simulink model "FullModelAddANN_Final_ANN_revised"  (R2024b)
settings: Solver=ode4  StartTime=0.0  StopTime=40  FixedStep=1e-5  RelTol=1e-3
values from neighbouring files (symbols this model uses):
  Dp = 2.506338228783948e3    (= 2506.33822878)    [FullModelAddANNm_Final.m]    (also in main_opal_ann_control.m)
  Dq = 1.033099625954584    (= 1.03309962595)    [FullModelAddANNm_Final.m]    (also in main_opal_ann_control.m)
  Kp = 0.006383815167581    (= 0.00638381516758)    [FullModelAddANNm_Final.m]    (also in main_opal_ann_control.m)
  Kq = 0.076670166944346    (= 0.0766701669443)    [FullModelAddANNm_Final.m]    (also in main_opal_ann_control.m)
undefined symbols (not defined in the file or in its folder): Filter, Ls, params
libraries: neural x88, spsCurrentMeasurementLib x6, spsParallelRLCBranchLib x6, spsIGBTDiodeLib x6, spsMeanLib x6, spsSeriesRLCBranchLib x6, simulink x4, spsVoltageMeasurementLib x4, spsVariableInductorLib x3, spsVariableResistorLib x3, spsDCVoltageSourceLib x1, spsThreePhaseSourceLib x1
(part 2 of 11)

== system FullModelAddANN_Final_ANN_revised/Feed-Forward Neural Network2/Process Output 1 ==
  a : Inport  PortDimensions=2
      mask Display: e = 0.06;c1 = [120 230 180]/255;c2 = ([120 230 180]+0)/(256+128);c3 = ([120 230 180]+128)/(256+128);patch([0 1 1 0],[0 0 1 1],c1);patch([0 1 1 1-e 1-e 0+e],[0 0 1 1-e 0+e 0+e],c2);patch([0 0 1 1-e 0+e 0+e],[0 1 1 1-e 1-e 0+e],c3);plot([0 1 1 0 0],[0 0 1 1 0]);
  mapminmax_reverse : neural/Processing Functions/mapminmax_reverse  xmin=[4.08518999999999987693399816635;0.100678000000000003599787135045]  xmax=[5.76843000000000039051428757375;1.28340000000000009627854069549]  ymin=-1  ymax=1
  y : Outport  PortDimensions=2
      mask Display: e = 0.06;c1 = [120 230 180]/255;c2 = ([120 230 180]+0)/(256+128);c3 = ([120 230 180]+128)/(256+128);patch([0 1 1 0],[0 0 1 1],c1);patch([0 1 1 1-e 1-e 0+e],[0 0 1 1-e 0+e 0+e],c2);patch([0 0 1 1-e 0+e 0+e],[0 1 1 1-e 1-e 0+e],c3);plot([0 1 1 0 0],[0 0 1 1 0]);
  wires:
  a/1 -> mapminmax_reverse/1
  mapminmax_reverse/1 -> y/1

== system FullModelAddANN_Final_ANN_revised/Feed-Forward Neural Network_Full/Layer 1 ==
  "p{1}" : Inport  PortDimensions=200
      mask Display: e = 0.06;c1 = [120 230 180]/255;c2 = ([120 230 180]+0)/(256+128);c3 = ([120 230 180]+128)/(256+128);patch([0 1 1 0],[0 0 1 1],c1);patch([0 1 1 1-e 1-e 0+e],[0 0 1 1-e 0+e 0+e],c2);patch([0 0 1 1-e 0+e 0+e],[0 1 1 1-e 1-e 0+e],c3);plot([0 1 1 0 0],[0 0 1 1 0]);
  Delays 1 : Subsystem
      mask Display: e = 0.06;c1 = [120 150 230]/255;c2 = ([120 150 230]+0)/383;c3 = ([120 150 230]+128)/383;patch([0 1 1 0],[0 0 1 1],c1);patch([0 1 1 1-e 1-e 0+e],[0 0 1 1-e 0+e 0+e],c2);patch([0 0 1 1-e 0+e 0+e],[0 1 1 1-e 1-e 0+e],c3);plot([0 1 1 0 0],[0 0 1 1 0]);disp('0');
  "IW{1,1}" : Subsystem
      mask Display: e = 0.06;c1 = [120 150 230]/255;c2 = ([120 150 230]+0)/383;c3 = ([120 150 230]+128)/383;patch([0 1 1 0],[0 0 1 1],c1);patch([0 1 1 1-e 1-e 0+e],[0 0 1 1-e 0+e 0+e],c2);patch([0 0 1 1-e 0+e 0+e],[0 1 1 1-e 1-e 0+e],c3);plot([0 1 1 0 0],[0 0 1 1 0]);disp('W');
  "b{1}" : Constant  Value=[-0.93745313626118720318203259012079797685146331787109375;-0.7522463014983509221877966410829685628414154052734375;0.7498310632798836916634854787844233214855194091796875;-0.448821782444379480114804437107522971928119659423828125;-0.56470000582433976799023866988136433064937591552734375;0.70695959761237425755808772009913809597492218017578125;0.305040499016989041791703130002133548259735107421875;0.045185602594992213543179104817681945860385894775390625;-0.385773129555622151798388586030341684818267822265625;0.402441364255973377250796829684986732900142669677734375;-0.458845318832768411798639363041729666292667388916015625;0.622328519648508216022264605271629989147186279296875;0.608199419849972944263072349713183939456939697265625;-0.7645386765801076567328209421248175203800201416015625;0.8420689862326191654773310801829211413860321044921875;-0.970352913386824500463490039692260324954986572265625]
      mask Display: e = 0.06;c1 = [120 150 230]/255;c2 = ([120 150 230]+0)/383;c3 = ([120 150 230]+128)/383;patch([0 1 1 0],[0 0 1 1],c1);patch([0 1 1 1-e 1-e 0+e],[0 0 1 1-e 0+e 0+e],c2);patch([0 0 1 1-e 0+e 0+e],[0 1 1 1-e 1-e 0+e],c3);plot([0 1 1 0 0],[0 0 1 1 0]);disp('b');
  netsum : Sum  Inputs=2  InputSameDT=on  SaturateOnIntegerOverflow=on  OutDataTypeStr=Inherit: Same as first input
      mask Display: e = 0.06;c1 = [120 150 230]/255;c2 = ([120 150 230]+0)/383;c3 = ([120 150 230]+128)/383;patch([0 1 1 0],[0 0 1 1],c1);patch([0 1 1 1-e 1-e 0+e],[0 0 1 1-e 0+e 0+e],c2);patch([0 0 1 1-e 0+e 0+e],[0 1 1 1-e 1-e 0+e],c3);plot([0 1 1 0 0],[0 0 1 1 0]);disp('+');
  tansig : neural/Transfer Functions/tansig
  "a{1}" : Outport  InitialOutput=[0;0;0;0;0;0;0;0;0;0;0;0;0;0;0;0]
      mask Display: e = 0.06;c1 = [120 230 180]/255;c2 = ([120 230 180]+0)/(256+128);c3 = ([120 230 180]+128)/(256+128);patch([0 1 1 0],[0 0 1 1],c1);patch([0 1 1 1-e 1-e 0+e],[0 0 1 1-e 0+e 0+e],c2);patch([0 0 1 1-e 0+e 0+e],[0 1 1 1-e 1-e 0+e],c3);plot([0 1 1 0 0],[0 0 1 1 0]);
  wires:
  "p{1}"/1 -> Delays 1/1("p{1}")
  Delays 1/1("pd{1,1}") -> "IW{1,1}"/1("pd{1,1}")
  "IW{1,1}"/1("iz{1,1}") -> netsum/1
  "b{1}"/1 -> netsum/2
  netsum/1 -> tansig/1
  tansig/1 -> "a{1}"/1

== system FullModelAddANN_Final_ANN_revised/Feed-Forward Neural Network_Full/Layer 2 ==
  "a{1} " : Inport  PortDimensions=16
      mask Display: e = 0.06;c1 = [120 230 180]/255;c2 = ([120 230 180]+0)/(256+128);c3 = ([120 230 180]+128)/(256+128);patch([0 1 1 0],[0 0 1 1],c1);patch([0 1 1 1-e 1-e 0+e],[0 0 1 1-e 0+e 0+e],c2);patch([0 0 1 1-e 0+e 0+e],[0 1 1 1-e 1-e 0+e],c3);plot([0 1 1 0 0],[0 0 1 1 0]);
  Delays 1 : Subsystem
      mask Display: e = 0.06;c1 = [120 150 230]/255;c2 = ([120 150 230]+0)/383;c3 = ([120 150 230]+128)/383;patch([0 1 1 0],[0 0 1 1],c1);patch([0 1 1 1-e 1-e 0+e],[0 0 1 1-e 0+e 0+e],c2);patch([0 0 1 1-e 0+e 0+e],[0 1 1 1-e 1-e 0+e],c3);plot([0 1 1 0 0],[0 0 1 1 0]);disp('0');
  "LW{2,1}" : Subsystem
      mask Display: e = 0.06;c1 = [120 150 230]/255;c2 = ([120 150 230]+0)/383;c3 = ([120 150 230]+128)/383;patch([0 1 1 0],[0 0 1 1],c1);patch([0 1 1 1-e 1-e 0+e],[0 0 1 1-e 0+e 0+e],c2);patch([0 0 1 1-e 0+e 0+e],[0 1 1 1-e 1-e 0+e],c3);plot([0 1 1 0 0],[0 0 1 1 0]);disp('W');
  "b{2}" : Constant  Value=[-0.349660820238201441867431640275754034519195556640625;0.1124855051162063634961896241293288767337799072265625]
      mask Display: e = 0.06;c1 = [120 150 230]/255;c2 = ([120 150 230]+0)/383;c3 = ([120 150 230]+128)/383;patch([0 1 1 0],[0 0 1 1],c1);patch([0 1 1 1-e 1-e 0+e],[0 0 1 1-e 0+e 0+e],c2);patch([0 0 1 1-e 0+e 0+e],[0 1 1 1-e 1-e 0+e],c3);plot([0 1 1 0 0],[0 0 1 1 0]);disp('b');
  netsum : Sum  Inputs=2  InputSameDT=on  SaturateOnIntegerOverflow=on  OutDataTypeStr=Inherit: Same as first input
      mask Display: e = 0.06;c1 = [120 150 230]/255;c2 = ([120 150 230]+0)/383;c3 = ([120 150 230]+128)/383;patch([0 1 1 0],[0 0 1 1],c1);patch([0 1 1 1-e 1-e 0+e],[0 0 1 1-e 0+e 0+e],c2);patch([0 0 1 1-e 0+e 0+e],[0 1 1 1-e 1-e 0+e],c3);plot([0 1 1 0 0],[0 0 1 1 0]);disp('+');
  purelin : neural/Transfer Functions/purelin
  "a{2}" : Outport  InitialOutput=[0;0]
      mask Display: e = 0.06;c1 = [120 230 180]/255;c2 = ([120 230 180]+0)/(256+128);c3 = ([120 230 180]+128)/(256+128);patch([0 1 1 0],[0 0 1 1],c1);patch([0 1 1 1-e 1-e 0+e],[0 0 1 1-e 0+e 0+e],c2);patch([0 0 1 1-e 0+e 0+e],[0 1 1 1-e 1-e 0+e],c3);plot([0 1 1 0 0],[0 0 1 1 0]);
  wires:
  "a{1} "/1 -> Delays 1/1("p{2}")
  Delays 1/1("pd{2,1}") -> "LW{2,1}"/1("ad{2,1}")
  "LW{2,1}"/1("lz{2,1}") -> netsum/1
  "b{2}"/1 -> netsum/2
  netsum/1 -> purelin/1
  purelin/1 -> "a{2}"/1

== system FullModelAddANN_Final_ANN_revised/Feed-Forward Neural Network_Full/Process Input 1 ==
  x : Inport  PortDimensions=200
      mask Display: e = 0.06;c1 = [120 230 180]/255;c2 = ([120 230 180]+0)/(256+128);c3 = ([120 230 180]+128)/(256+128);patch([0 1 1 0],[0 0 1 1],c1);patch([0 1 1 1-e 1-e 0+e],[0 0 1 1-e 0+e 0+e],c2);patch([0 0 1 1-e 0+e 0+e],[0 1 1 1-e 1-e 0+e],c3);plot([0 1 1 0 0],[0 0 1 1 0]);
  mapminmax : neural/Processing Functions/mapminmax  xmin=[-18.1541999999999994486188370502;-7.44869999999999965467623042059;3.20396999999999998465227690758;15.3264999999999993463006831007;26.545400000000000773070496507;39.4832999999999998408384271897;51.2171999999999982833287504036;62.2657999999999987039700499736;74.1317999999999983629095368087;85.9979000000000013415046851151;90.0867999999999966576069709845;84.7300000000000039790393202566;79.158100000000004570210876409;71.0503999999999962255969876423;70.2383999999999986130205797963;63.514400000000001966782292584;53.7342000000000012960299500264;49.1422999999999987608134688344;37.9063000000000016598278307356;33.1124999999999971578290569596;24.1713999999999984424903232139;20.1130999999999993121946317842;18.4002000000000016655121726217;7.66408000000000022566837287741;0.2774440000000000239310793404;-7.13638999999999956713736537495;-7.5049000000000001264766069653;-11.9069000000000002614797267597;-24.4015999999999984026999300113;-28.9071999999999995623056747718;-36.3990999999999971237230056431;-44.7280000000000015347723092418;-51.1516000000000019554136088118;-60.0354999999999989768184605055;-67.1332000000000022055246517994;-72.0875000000000056843418860808;-72.9534000000000020236257114448;-78.9898000000000024556356947869;-86.867500000000006821210263297;-90.046999999999997044142219238;-95.992500000000006821210263297;-96.6642999999999972260411595926;-100.924000000000006593836587854;-100.814999999999997726263245568;-103.352999999999994429344951641;-106.415000000000006252776074689;-105.480000000000003979039320257;-108.036000000000001364242052659;-108.385999999999995679900166579;-113.061999999999997612576407846;-113.593999999999994088284438476;-113.680999999999997385202732403;-113.947999999999993292476574425;-117.102999999999994429344951641;-118.498000000000004661160346586;-126.837000000000003296918293927;-137.923000000000001818989403546;-145.596000000000003637978807092;-149.325999999999993406163412146;-160.45699999999999363353708759;-169.43899999999999295141606126;-170.971000000000003637978807092;-175.950999999999993406163412146;-177.468999999999994088284438476;-177.054000000000002046363078989;-193.711999999999989086063578725;-190.943999999999988403942552395;-200.5;-204.413000000000010913936421275;-206.586999999999989086063578725;-212.259999999999990905052982271;-214.850999999999999090505298227;-215.110000000000013642420526594;-219.927999999999997271515894681;-213.552999999999997271515894681;-210.719999999999998863131622784;-204.14300000000000068212102633;-199.899000000000000909494701773;-194.169000000000011141310096718;-190.197000000000002728484105319;-187.044999999999987494447850622;-184.040999999999996816768543795;-184.417000000000001591615728103;-181.421999999999997044142219238;-173.832999999999998408384271897;-167.014999999999986357579473406;-159.828000000000002955857780762;-144.580000000000012505552149378;-132.871000000000009322320693173;-122.415999999999996816768543795;-110.460999999999998522071109619;-92.6098000000000070031092036515;-79.2937000000000011823431123048;-66.6076000000000050249582272954;-55.4363000000000027966962079518;-46.4945999999999983742782205809;-40.2008999999999971919351082761;-30.580400000000000915179043659;-26.3471000000000010743406164693;-23.6697999999999986187049216824;-12.1233000000000004092726157978;-12.2150999999999996248334355187;-12.7461999999999999744204615126;-12.8681000000000000937916411203;-13.8106000000000008753886504564;-13.5084999999999997299937604112;-12.3736999999999994770405464806;-11.4261999999999996902033672086;-10.8213000000000008071765478235;-9.86029000000000088732576841721;-8.03398999999999929855221125763;-5.84081000000000027938540370087;-4.18013999999999974477304931497;-2.83502000000000009549694368616;-1.46507999999999993789856489457;0.335683999999999982399856435222;1.85640000000000005009326287109;3.5641500000000001513456027169;4.22681000000000040017766878009;2.03202000000000015944578990457;-0.313620999999999983121057312019;-2.61730000000000018189894035459;-5.01956999999999986528109729989 ...(+2532 chars)]  xmax=[112.79999999999999715782905696;111.144999999999996020960679743;115.558000000000006934897101019;117.849000000000003751665644813;122.192999999999997839950083289;127.019999999999996020960679743;136.147999999999996134647517465;144.45699999999999363353708759;152.650000000000005684341886081;158.165999999999996816768543795;164.931000000000011596057447605;171.423000000000001818989403546;174.419999999999987494447850622;175.741000000000013869794202037;178.253999999999990677679306827;190.344999999999998863131622784;192.007000000000005002220859751;203.405000000000001136868377216;200.974999999999994315658113919;205.979999999999989768184605055;214.807999999999992724042385817;214.694999999999993178789736703;213.953000000000002955857780762;217.332999999999998408384271897;213;210.046999999999997044142219238;206.548000000000001818989403546;199.008000000000009777068044059;193.161000000000001364242052659;190.629999999999995452526491135;186.881000000000000227373675443;185.817000000000007275957614183;183.401999999999986812326824293;181.348999999999989540810929611;175.411000000000001364242052659;167.467000000000012960299500264;165.415999999999996816768543795;147.104999999999989768184605055;132.336999999999989086063578725;119.719999999999998863131622784;106.367000000000004433786671143;94.7475000000000022737367544323;78.5541000000000053660187404603;66.109499999999997044142219238;55.6694000000000031036506698001;47.8620999999999980900611262769;39.058199999999999363353708759;31.5702999999999995850430423161;27.5088000000000008071765478235;22.4850999999999991985077940626;14.745699999999999363353708759;6.72907999999999972828845784534;-2.79722999999999988318677424104;-15.5510000000000001563194018672;-25.9831000000000003069544618484;-39.7043000000000034788172342815;-51.9249000000000009436007530894;-62.2948999999999983856469043531;-74.8230999999999966121322358958;-85.0691999999999950432538753375;-81.6354000000000041836756281555;-79.7052999999999940428097033873;-75.7283000000000043883119360544;-65.9572000000000002728484105319;-60.3667999999999977944753482006;-55.1897999999999981923792802263;-49.7203999999999979308995534666;-43.0686999999999997612576407846;-38.2561999999999997612576407846;-31.8615999999999992553512129234;-26.1017000000000010118128557224;-20.3201000000000000511590769747;-13.9556000000000004490630090004;-3.78928000000000020364154806884;0.792328000000000032265745630866;8.75453000000000081115558714373;12.4443999999999999062083588797;12.5769000000000001904254531837;25.1676999999999999602096067974;30.4983000000000004092726157978;41.3939999999999983515408530366;49.8380000000000009663381206337;54.6548000000000016029844118748;61.4352000000000018076207197737;68.6329000000000064574123825878;77.1235999999999961573848850094;84.3909000000000020236257114448;87.9608999999999952024154481478;90.2530000000000001136868377216;95.6707999999999998408384271897;96.7533999999999991814547684044;99.2844999999999942019712761976;101.617999999999994997779140249;102.167000000000001591615728103;106.757000000000005002220859751;111.489999999999994884092302527;110.766000000000005343281372916;113.855999999999994543031789362;113.308999999999997498889570124;112.527000000000001023181539495;52.6158000000000001250555214938;51.8245000000000004547473508865;50.9217000000000012960299500264;49.8179000000000016257217794191;48.5294999999999987494447850622;47.0690999999999988290255714674;45.4183000000000021145751816221;43.5947999999999993292476574425;41.6131999999999990791366144549;39.4806000000000025806912162807;37.1856000000000008753886504564;37.7886999999999986243892635684;38.4459000000000017394086171407;38.670400000000000773070496507;38.4410000000000025011104298756;38.3459000000000003183231456205;38.2884000000000028762769943569;37.8397000000000005570655048359;36.9037999999999968281372275669;35.9100999999999999090505298227;34.9179000000000030468072509393;33.7860000000000013642420526594;32.5932999999999992724042385817;31.6207999999999991302956914296;30.511500000000001620037437533 ...(+2402 chars)]  ymin=-1  ymax=1
  p : Outport  PortDimensions=200
      mask Display: e = 0.06;c1 = [120 230 180]/255;c2 = ([120 230 180]+0)/(256+128);c3 = ([120 230 180]+128)/(256+128);patch([0 1 1 0],[0 0 1 1],c1);patch([0 1 1 1-e 1-e 0+e],[0 0 1 1-e 0+e 0+e],c2);patch([0 0 1 1-e 0+e 0+e],[0 1 1 1-e 1-e 0+e],c3);plot([0 1 1 0 0],[0 0 1 1 0]);
  wires:
  x/1 -> mapminmax/1
  mapminmax/1 -> p/1

== system FullModelAddANN_Final_ANN_revised/Feed-Forward Neural Network_Full/Process Output 1 ==
  a : Inport  PortDimensions=2
      mask Display: e = 0.06;c1 = [120 230 180]/255;c2 = ([120 230 180]+0)/(256+128);c3 = ([120 230 180]+128)/(256+128);patch([0 1 1 0],[0 0 1 1],c1);patch([0 1 1 1-e 1-e 0+e],[0 0 1 1-e 0+e 0+e],c2);patch([0 0 1 1-e 0+e 0+e],[0 1 1 1-e 1-e 0+e],c3);plot([0 1 1 0 0],[0 0 1 1 0]);
  mapminmax_reverse : neural/Processing Functions/mapminmax_reverse  xmin=[1.08938000000000001499245172454;0.0344836000000000031384672638524]  xmax=[11.5252999999999996560973158921;2.56680000000000019255708139099]  ymin=-1  ymax=1
  y : Outport  PortDimensions=2
      mask Display: e = 0.06;c1 = [120 230 180]/255;c2 = ([120 230 180]+0)/(256+128);c3 = ([120 230 180]+128)/(256+128);patch([0 1 1 0],[0 0 1 1],c1);patch([0 1 1 1-e 1-e 0+e],[0 0 1 1-e 0+e 0+e],c2);patch([0 0 1 1-e 0+e 0+e],[0 1 1 1-e 1-e 0+e],c3);plot([0 1 1 0 0],[0 0 1 1 0]);
  wires:
  a/1 -> mapminmax_reverse/1
  mapminmax_reverse/1 -> y/1

== system FullModelAddANN_Final_ANN_revised/Feed-Forward Neural Network_RealTime/Layer 1 ==
  "p{1}" : Inport  PortDimensions=200
      mask Display: e = 0.06;c1 = [120 230 180]/255;c2 = ([120 230 180]+0)/(256+128);c3 = ([120 230 180]+128)/(256+128);patch([0 1 1 0],[0 0 1 1],c1);patch([0 1 1 1-e 1-e 0+e],[0 0 1 1-e 0+e 0+e],c2);patch([0 0 1 1-e 0+e 0+e],[0 1 1 1-e 1-e 0+e],c3);plot([0 1 1 0 0],[0 0 1 1 0]);
  Delays 1 : Subsystem
      mask Display: e = 0.06;c1 = [120 150 230]/255;c2 = ([120 150 230]+0)/383;c3 = ([120 150 230]+128)/383;patch([0 1 1 0],[0 0 1 1],c1);patch([0 1 1 1-e 1-e 0+e],[0 0 1 1-e 0+e 0+e],c2);patch([0 0 1 1-e 0+e 0+e],[0 1 1 1-e 1-e 0+e],c3);plot([0 1 1 0 0],[0 0 1 1 0]);disp('0');
  "IW{1,1}" : Subsystem
      mask Display: e = 0.06;c1 = [120 150 230]/255;c2 = ([120 150 230]+0)/383;c3 = ([120 150 230]+128)/383;patch([0 1 1 0],[0 0 1 1],c1);patch([0 1 1 1-e 1-e 0+e],[0 0 1 1-e 0+e 0+e],c2);patch([0 0 1 1-e 0+e 0+e],[0 1 1 1-e 1-e 0+e],c3);plot([0 1 1 0 0],[0 0 1 1 0]);disp('W');
  "b{1}" : Constant  Value=[-0.7049546789635818822006285699899308383464813232421875;-0.53176379998661749137767174033797346055507659912109375;0.56664598808941513130577050105785019695758819580078125;-0.1546177681597955544390288196154870092868804931640625;-0.2268178266264400944063339693457237444818019866943359375;0.222921193941614304012688307921052910387516021728515625;0.139048173582270673254157600240432657301425933837890625;-0.1366552484170819592446122214823844842612743377685546875;0.0964330208189879412028489014119259081780910491943359375;-0.04916039248471136546836390834869234822690486907958984375;-0.7305750372192016950378956607892177999019622802734375;-0.1797210239748362747835841446431004442274570465087890625;0.45485073167759104695306859866832382977008819580078125;-0.475714928798503411400133700226433575153350830078125;0.77984233044243456145494519660132937133312225341796875;-0.73985496629634706078348926894250325858592987060546875]
      mask Display: e = 0.06;c1 = [120 150 230]/255;c2 = ([120 150 230]+0)/383;c3 = ([120 150 230]+128)/383;patch([0 1 1 0],[0 0 1 1],c1);patch([0 1 1 1-e 1-e 0+e],[0 0 1 1-e 0+e 0+e],c2);patch([0 0 1 1-e 0+e 0+e],[0 1 1 1-e 1-e 0+e],c3);plot([0 1 1 0 0],[0 0 1 1 0]);disp('b');
  netsum : Sum  Inputs=2  InputSameDT=on  SaturateOnIntegerOverflow=on  OutDataTypeStr=Inherit: Same as first input
      mask Display: e = 0.06;c1 = [120 150 230]/255;c2 = ([120 150 230]+0)/383;c3 = ([120 150 230]+128)/383;patch([0 1 1 0],[0 0 1 1],c1);patch([0 1 1 1-e 1-e 0+e],[0 0 1 1-e 0+e 0+e],c2);patch([0 0 1 1-e 0+e 0+e],[0 1 1 1-e 1-e 0+e],c3);plot([0 1 1 0 0],[0 0 1 1 0]);disp('+');
  tansig : neural/Transfer Functions/tansig
  "a{1}" : Outport  InitialOutput=[0;0;0;0;0;0;0;0;0;0;0;0;0;0;0;0]
      mask Display: e = 0.06;c1 = [120 230 180]/255;c2 = ([120 230 180]+0)/(256+128);c3 = ([120 230 180]+128)/(256+128);patch([0 1 1 0],[0 0 1 1],c1);patch([0 1 1 1-e 1-e 0+e],[0 0 1 1-e 0+e 0+e],c2);patch([0 0 1 1-e 0+e 0+e],[0 1 1 1-e 1-e 0+e],c3);plot([0 1 1 0 0],[0 0 1 1 0]);
  wires:
  "p{1}"/1 -> Delays 1/1("p{1}")
  Delays 1/1("pd{1,1}") -> "IW{1,1}"/1("pd{1,1}")
  "IW{1,1}"/1("iz{1,1}") -> netsum/1
  "b{1}"/1 -> netsum/2
  netsum/1 -> tansig/1
  tansig/1 -> "a{1}"/1

== system FullModelAddANN_Final_ANN_revised/Feed-Forward Neural Network_RealTime/Layer 2 ==
  "a{1} " : Inport  PortDimensions=16
      mask Display: e = 0.06;c1 = [120 230 180]/255;c2 = ([120 230 180]+0)/(256+128);c3 = ([120 230 180]+128)/(256+128);patch([0 1 1 0],[0 0 1 1],c1);patch([0 1 1 1-e 1-e 0+e],[0 0 1 1-e 0+e 0+e],c2);patch([0 0 1 1-e 0+e 0+e],[0 1 1 1-e 1-e 0+e],c3);plot([0 1 1 0 0],[0 0 1 1 0]);
  Delays 1 : Subsystem
      mask Display: e = 0.06;c1 = [120 150 230]/255;c2 = ([120 150 230]+0)/383;c3 = ([120 150 230]+128)/383;patch([0 1 1 0],[0 0 1 1],c1);patch([0 1 1 1-e 1-e 0+e],[0 0 1 1-e 0+e 0+e],c2);patch([0 0 1 1-e 0+e 0+e],[0 1 1 1-e 1-e 0+e],c3);plot([0 1 1 0 0],[0 0 1 1 0]);disp('0');
  "LW{2,1}" : Subsystem
      mask Display: e = 0.06;c1 = [120 150 230]/255;c2 = ([120 150 230]+0)/383;c3 = ([120 150 230]+128)/383;patch([0 1 1 0],[0 0 1 1],c1);patch([0 1 1 1-e 1-e 0+e],[0 0 1 1-e 0+e 0+e],c2);patch([0 0 1 1-e 0+e 0+e],[0 1 1 1-e 1-e 0+e],c3);plot([0 1 1 0 0],[0 0 1 1 0]);disp('W');
  "b{2}" : Constant  Value=[-0.78120311102570483274831758535583503544330596923828125;0.0785637733916535740963382750123855657875537872314453125]
      mask Display: e = 0.06;c1 = [120 150 230]/255;c2 = ([120 150 230]+0)/383;c3 = ([120 150 230]+128)/383;patch([0 1 1 0],[0 0 1 1],c1);patch([0 1 1 1-e 1-e 0+e],[0 0 1 1-e 0+e 0+e],c2);patch([0 0 1 1-e 0+e 0+e],[0 1 1 1-e 1-e 0+e],c3);plot([0 1 1 0 0],[0 0 1 1 0]);disp('b');
  netsum : Sum  Inputs=2  InputSameDT=on  SaturateOnIntegerOverflow=on  OutDataTypeStr=Inherit: Same as first input
      mask Display: e = 0.06;c1 = [120 150 230]/255;c2 = ([120 150 230]+0)/383;c3 = ([120 150 230]+128)/383;patch([0 1 1 0],[0 0 1 1],c1);patch([0 1 1 1-e 1-e 0+e],[0 0 1 1-e 0+e 0+e],c2);patch([0 0 1 1-e 0+e 0+e],[0 1 1 1-e 1-e 0+e],c3);plot([0 1 1 0 0],[0 0 1 1 0]);disp('+');
  purelin : neural/Transfer Functions/purelin
  "a{2}" : Outport  InitialOutput=[0;0]
      mask Display: e = 0.06;c1 = [120 230 180]/255;c2 = ([120 230 180]+0)/(256+128);c3 = ([120 230 180]+128)/(256+128);patch([0 1 1 0],[0 0 1 1],c1);patch([0 1 1 1-e 1-e 0+e],[0 0 1 1-e 0+e 0+e],c2);patch([0 0 1 1-e 0+e 0+e],[0 1 1 1-e 1-e 0+e],c3);plot([0 1 1 0 0],[0 0 1 1 0]);
  wires:
  "a{1} "/1 -> Delays 1/1("p{2}")
  Delays 1/1("pd{2,1}") -> "LW{2,1}"/1("ad{2,1}")
  "LW{2,1}"/1("lz{2,1}") -> netsum/1
  "b{2}"/1 -> netsum/2
  netsum/1 -> purelin/1
  purelin/1 -> "a{2}"/1

== system FullModelAddANN_Final_ANN_revised/Feed-Forward Neural Network_RealTime/Process Input 1 ==
  x : Inport  PortDimensions=200
      mask Display: e = 0.06;c1 = [120 230 180]/255;c2 = ([120 230 180]+0)/(256+128);c3 = ([120 230 180]+128)/(256+128);patch([0 1 1 0],[0 0 1 1],c1);patch([0 1 1 1-e 1-e 0+e],[0 0 1 1-e 0+e 0+e],c2);patch([0 0 1 1-e 0+e 0+e],[0 1 1 1-e 1-e 0+e],c3);plot([0 1 1 0 0],[0 0 1 1 0]);
  mapminmax : neural/Processing Functions/mapminmax  xmin=[-17.0536999999999991928234521765;-6.90960000000000018616219676915;1.32868000000000008320455435751;12.5934000000000008157030606526;26.8697000000000016939338820521;41.5780999999999991700860846322;53.7240999999999999658939486835;67.3171999999999997044142219238;78.8409999999999939745976007544;88.2877000000000009549694368616;87.0142000000000024328983272426;83.9624000000000023646862246096;75.1424999999999982946974341758;70.2459000000000060026650317013;61.7374000000000009436007530894;57.8691999999999993065102898981;52.2186999999999983401721692644;44.6687000000000011823431123048;39.1567999999999969418240652885;34.2475999999999984879650583025;24.8386999999999993349319993285;21.4954000000000000625277607469;15.5536999999999991928234521765;6.39240999999999992553512129234;2.04654999999999986926013662014;-1.18479000000000000980548975349;-8.32602999999999937585926090833;-16.5778999999999996362021192908;-21.2610999999999989995558280498;-28.4237999999999999545252649114;-36.734499999999997044142219238;-41.9243999999999985561771609355;-51.339199999999998169641912682;-60.2991000000000028080648917239;-64.033100000000004570210876409;-70.556600000000003092281986028;-75.6507000000000005002220859751;-81.1367000000000047066350816749;-86.5153999999999996362021192908;-88.4420999999999963847585604526;-95.1997000000000070940586738288;-95.5378999999999933834260446019;-99.909199999999998453859006986;-101.362999999999999545252649114;-102.371999999999999886313162278;-105.39300000000000068212102633;-108.334999999999993747223925311;-107.676000000000001932676241267;-106.683000000000006934897101019;-112.131000000000000227373675443;-110.46800000000000352429196937;-110.873000000000004661160346586;-110.787000000000006139089236967;-112.980000000000003979039320257;-111.801000000000001932676241267;-116.733999999999994656718627084;-124.862999999999999545252649114;-132.080999999999988858689903282;-139.818999999999988403942552395;-149.477000000000003865352482535;-155.419000000000011141310096718;-162.912000000000006139089236967;-172.710000000000007958078640513;-174.960000000000007958078640513;-176.641999999999995907273842022;-175.318000000000012050804798491;-172.590000000000003410605131648;-175.985000000000013642420526594;-178.417000000000001591615728103;-178.522999999999996134647517465;-183.858000000000004092726157978;-183.539999999999992041921359487;-183.884999999999990905052982271;-186.243999999999999772626324557;-186.263000000000005229594535194;-188.723999999999989540810929611;-184.569999999999993178789736703;-181.26800000000000068212102633;-179.665999999999996816768543795;-178.229999999999989768184605055;-176.842999999999989313437254168;-174.032999999999987039700499736;-173.526999999999986812326824293;-173.508000000000009777068044059;-171.633000000000009777068044059;-165.169000000000011141310096718;-155.799000000000006593836587854;-143.864000000000004320099833421;-131.848999999999989540810929611;-120.766999999999995907273842022;-109.695999999999997953636921011;-96.5019999999999953388396534137;-81.3294000000000067984728957526;-68.0889999999999986357579473406;-56.1655000000000015347723092418;-46.9710999999999998522071109619;-36.5542000000000015802470443305;-32.4759999999999990905052982271;-25.1271999999999984254372975556;-22.5638000000000005229594535194;-9.98273999999999972487785271369;-9.56886000000000080945028457791;-9.52431999999999945316631055903;-9.33891999999999988801846484421;-9.18894000000000055194959713845;-8.80775000000000041211478674086;-8.24868000000000023419488570653;-7.54786000000000001364242052659;-6.74500000000000010658141036402;-5.84464000000000005741185304942;-4.75785999999999997811528373859;-3.56252000000000013102408047416;-2.2542399999999997994848399685;-1.2108600000000000473932004752;-0.556723999999999996646238287212;0.0785335000000000060804694612671;1.04598999999999997534416706912;2.32660000000000000142108547152;3.49752999999999980573761604319;4.31245999999999973795183905168;0.123700000000000004396483177516;-4.44273000000000006792788553867 ...(+2569 chars)]  xmax=[111.865999999999999658939486835;112.992000000000004433786671143;112.234999999999999431565811392;114.799000000000006593836587854;113.064999999999997726263245568;118.135999999999995679900166579;124.359999999999999431565811392;132.878999999999990677679306827;140.645000000000010231815394945;148.348000000000013187673175707;156.0970000000000084128259914;164.181000000000011596057447605;170.609000000000008867573342286;175.45699999999999363353708759;177.248999999999995225152815692;173.300000000000011368683772162;173.352000000000003865352482535;175.931000000000011596057447605;176.426999999999992496668710373;179.361999999999994770405464806;179.365000000000009094947017729;179.772999999999996134647517465;184.776999999999986812326824293;185.591000000000008185452315956;185.283999999999991814547684044;183.663999999999987267074175179;183.818999999999988403942552395;182.574999999999988631316227838;180.169000000000011141310096718;177.211000000000012732925824821;175.573000000000007503331289627;175.9720000000000084128259914;174.123999999999995225152815692;172.474999999999994315658113919;170.62200000000001409716787748;166.653999999999996362021192908;156.840000000000003410605131648;146.054000000000002046363078989;132.260999999999995679900166579;121.527000000000001023181539495;107.483999999999994656718627084;96.5798000000000058662408264354;80.6736999999999966348696034402;67.5002999999999957481122692116;55.3132999999999981355358613655;46.9207999999999998408384271897;35.5009000000000014551915228367;31.0551999999999992496668710373;25.0103000000000008640199666843;24.5443999999999995509369909996;19.8542999999999985050180839607;6.81196000000000001506350599811;-1.50009999999999998898658759572;-14.6496999999999992780885804677;-28.0711000000000012732925824821;-43.2413000000000025124791136477;-56.7535000000000025011104298756;-67.7192000000000007275957614183;-77.1479999999999961346475174651;-89.4813999999999936107997200452;-84.8738000000000027966962079518;-79.4834000000000031604940886609;-70.8067000000000064119376474991;-64.3097999999999956344254314899;-64.0426999999999964074959279969;-54.8742999999999980786924425047;-44.1308000000000006934897101019;-40.21529999999999915871740086;-34.423099999999998033217707416;-27.5173999999999985277554515051;-18.9917000000000015802470443305;-12.0957000000000007844391802792;-8.20207000000000086004092736403;-4.99021999999999987807086654357;2.17446999999999990293986229517;6.72055999999999986727061696001;12.6120000000000000994759830064;21.4647000000000005570655048359;28.8947000000000002728484105319;36.8487000000000008981260180008;42.3740999999999985448084771633;48.3299000000000020804691303056;57.7278999999999982151166477706;61.9328999999999965098140819464;69.3426000000000044565240386873;76.7212999999999993860910763033;82.5904000000000024783730623312;86.4916000000000053660187404603;88.1903999999999967940311762504;91.5768000000000057525539887138;95.8619999999999947704054648057;99.7070999999999969531927490607;103.042000000000001591615728103;105.320999999999997953636921011;108.423000000000001818989403546;107.277000000000001023181539495;107.939999999999997726263245568;111.680000000000006821210263297;112.150999999999996248334355187;113.51800000000000068212102633;104.658000000000001250555214938;103.278999999999996362021192908;101.56100000000000704858393874;99.7075999999999993406163412146;97.511200000000002319211489521;94.7877000000000009549694368616;91.5193000000000012050804798491;87.9523999999999972487785271369;84.0852000000000003865352482535;79.8438000000000016598278307356;75.1761000000000052523319027387;70.2203999999999979308995534666;64.9583999999999974761522025801;59.4846000000000003637978807092;53.7462000000000017507773009129;47.5636999999999972033037920482;44.7411000000000029785951483063;43.2085000000000007958078640513;41.4568999999999974193087837193;39.5840000000000031832314562052;37.5833999999999974761522025801;35.4305999999999983174348017201;33.1876000000000033196556614712;32.280999999999998806288203923 ...(+2433 chars)]  ymin=-1  ymax=1
  p : Outport  PortDimensions=200
      mask Display: e = 0.06;c1 = [120 230 180]/255;c2 = ([120 230 180]+0)/(256+128);c3 = ([120 230 180]+128)/(256+128);patch([0 1 1 0],[0 0 1 1],c1);patch([0 1 1 1-e 1-e 0+e],[0 0 1 1-e 0+e 0+e],c2);patch([0 0 1 1-e 0+e 0+e],[0 1 1 1-e 1-e 0+e],c3);plot([0 1 1 0 0],[0 0 1 1 0]);
  wires:
  x/1 -> mapminmax/1
  mapminmax/1 -> p/1

== system FullModelAddANN_Final_ANN_revised/Feed-Forward Neural Network_RealTime/Process Output 1 ==
  a : Inport  PortDimensions=2
      mask Display: e = 0.06;c1 = [120 230 180]/255;c2 = ([120 230 180]+0)/(256+128);c3 = ([120 230 180]+128)/(256+128);patch([0 1 1 0],[0 0 1 1],c1);patch([0 1 1 1-e 1-e 0+e],[0 0 1 1-e 0+e 0+e],c2);patch([0 0 1 1-e 0+e 0+e],[0 1 1 1-e 1-e 0+e],c3);plot([0 1 1 0 0],[0 0 1 1 0]);
  mapminmax_reverse : neural/Processing Functions/mapminmax_reverse  xmin=[1.77370000000000005435651928565;0.0371483000000000021523227644593]  xmax=[11.5290999999999996816768543795;1.28340000000000009627854069549]  ymin=-1  ymax=1
  y : Outport  PortDimensions=2
      mask Display: e = 0.06;c1 = [120 230 180]/255;c2 = ([120 230 180]+0)/(256+128);c3 = ([120 230 180]+128)/(256+128);patch([0 1 1 0],[0 0 1 1],c1);patch([0 1 1 1-e 1-e 0+e],[0 0 1 1-e 0+e 0+e],c2);patch([0 0 1 1-e 0+e 0+e],[0 1 1 1-e 1-e 0+e],c3);plot([0 1 1 0 0],[0 0 1 1 0]);
  wires:
  a/1 -> mapminmax_reverse/1
  mapminmax_reverse/1 -> y/1

== system FullModelAddANN_Final_ANN_revised/Feed-Forward Neural Network_strength/Layer 1 ==
  "p{1}" : Inport  PortDimensions=200
      mask Display: e = 0.06;c1 = [120 230 180]/255;c2 = ([120 230 180]+0)/(256+128);c3 = ([120 230 180]+128)/(256+128);patch([0 1 1 0],[0 0 1 1],c1);patch([0 1 1 1-e 1-e 0+e],[0 0 1 1-e 0+e 0+e],c2);patch([0 0 1 1-e 0+e 0+e],[0 1 1 1-e 1-e 0+e],c3);plot([0 1 1 0 0],[0 0 1 1 0]);
  Delays 1 : Subsystem
      mask Display: e = 0.06;c1 = [120 150 230]/255;c2 = ([120 150 230]+0)/383;c3 = ([120 150 230]+128)/383;patch([0 1 1 0],[0 0 1 1],c1);patch([0 1 1 1-e 1-e 0+e],[0 0 1 1-e 0+e 0+e],c2);patch([0 0 1 1-e 0+e 0+e],[0 1 1 1-e 1-e 0+e],c3);plot([0 1 1 0 0],[0 0 1 1 0]);disp('0');
  "IW{1,1}" : Subsystem
      mask Display: e = 0.06;c1 = [120 150 230]/255;c2 = ([120 150 230]+0)/383;c3 = ([120 150 230]+128)/383;patch([0 1 1 0],[0 0 1 1],c1);patch([0 1 1 1-e 1-e 0+e],[0 0 1 1-e 0+e 0+e],c2);patch([0 0 1 1-e 0+e 0+e],[0 1 1 1-e 1-e 0+e],c3);plot([0 1 1 0 0],[0 0 1 1 0]);disp('W');
  "b{1}" : Constant  Value=[-0.51942642685148732173416874502436257898807525634765625;-0.404648297130346890071450616233050823211669921875;0.443234607163469351842621790638077072799205780029296875;-0.27862991561518624106241759363911114633083343505859375;-0.203628983251990025582500720702228136360645294189453125;0.1016980160758019502420523849650635384023189544677734375;0.16493317679162278199811453305301256477832794189453125;-0.00896299740757437214677683101626826100982725620269775390625;0.07529216472706588836327767921829945407807826995849609375;0.08530217140173239342981759136819164268672466278076171875;-0.1951501613926993339287463413711520843207836151123046875;0.345828663945776881849525352663476951420307159423828125;0.292598628128426074823664748691953718662261962890625;-0.363644119784108099668884506172616966068744659423828125;0.435223097900301503226927479772712104022502899169921875;-0.5313207864293183479986737438593991100788116455078125]
      mask Display: e = 0.06;c1 = [120 150 230]/255;c2 = ([120 150 230]+0)/383;c3 = ([120 150 230]+128)/383;patch([0 1 1 0],[0 0 1 1],c1);patch([0 1 1 1-e 1-e 0+e],[0 0 1 1-e 0+e 0+e],c2);patch([0 0 1 1-e 0+e 0+e],[0 1 1 1-e 1-e 0+e],c3);plot([0 1 1 0 0],[0 0 1 1 0]);disp('b');
  netsum : Sum  Inputs=2  InputSameDT=on  SaturateOnIntegerOverflow=on  OutDataTypeStr=Inherit: Same as first input
      mask Display: e = 0.06;c1 = [120 150 230]/255;c2 = ([120 150 230]+0)/383;c3 = ([120 150 230]+128)/383;patch([0 1 1 0],[0 0 1 1],c1);patch([0 1 1 1-e 1-e 0+e],[0 0 1 1-e 0+e 0+e],c2);patch([0 0 1 1-e 0+e 0+e],[0 1 1 1-e 1-e 0+e],c3);plot([0 1 1 0 0],[0 0 1 1 0]);disp('+');
  tansig : neural/Transfer Functions/tansig
  "a{1}" : Outport  InitialOutput=[0;0;0;0;0;0;0;0;0;0;0;0;0;0;0;0]
      mask Display: e = 0.06;c1 = [120 230 180]/255;c2 = ([120 230 180]+0)/(256+128);c3 = ([120 230 180]+128)/(256+128);patch([0 1 1 0],[0 0 1 1],c1);patch([0 1 1 1-e 1-e 0+e],[0 0 1 1-e 0+e 0+e],c2);patch([0 0 1 1-e 0+e 0+e],[0 1 1 1-e 1-e 0+e],c3);plot([0 1 1 0 0],[0 0 1 1 0]);
  wires:
  "p{1}"/1 -> Delays 1/1("p{1}")
  Delays 1/1("pd{1,1}") -> "IW{1,1}"/1("pd{1,1}")
  "IW{1,1}"/1("iz{1,1}") -> netsum/1
  "b{1}"/1 -> netsum/2
  netsum/1 -> tansig/1
  tansig/1 -> "a{1}"/1

== system FullModelAddANN_Final_ANN_revised/Feed-Forward Neural Network_strength/Layer 2 ==
  "a{1} " : Inport  PortDimensions=16
      mask Display: e = 0.06;c1 = [120 230 180]/255;c2 = ([120 230 180]+0)/(256+128);c3 = ([120 230 180]+128)/(256+128);patch([0 1 1 0],[0 0 1 1],c1);patch([0 1 1 1-e 1-e 0+e],[0 0 1 1-e 0+e 0+e],c2);patch([0 0 1 1-e 0+e 0+e],[0 1 1 1-e 1-e 0+e],c3);plot([0 1 1 0 0],[0 0 1 1 0]);
  Delays 1 : Subsystem
      mask Display: e = 0.06;c1 = [120 150 230]/255;c2 = ([120 150 230]+0)/383;c3 = ([120 150 230]+128)/383;patch([0 1 1 0],[0 0 1 1],c1);patch([0 1 1 1-e 1-e 0+e],[0 0 1 1-e 0+e 0+e],c2);patch([0 0 1 1-e 0+e 0+e],[0 1 1 1-e 1-e 0+e],c3);plot([0 1 1 0 0],[0 0 1 1 0]);disp('0');
  "LW{2,1}" : Subsystem
      mask Display: e = 0.06;c1 = [120 150 230]/255;c2 = ([120 150 230]+0)/383;c3 = ([120 150 230]+128)/383;patch([0 1 1 0],[0 0 1 1],c1);patch([0 1 1 1-e 1-e 0+e],[0 0 1 1-e 0+e 0+e],c2);patch([0 0 1 1-e 0+e 0+e],[0 1 1 1-e 1-e 0+e],c3);plot([0 1 1 0 0],[0 0 1 1 0]);disp('W');
  "b{2}" : Constant  Value=[-0.038751620189991474452195774347273982129991054534912109375;0.01461393464810432051004251974291037186048924922943115234375]
      mask Display: e = 0.06;c1 = [120 150 230]/255;c2 = ([120 150 230]+0)/383;c3 = ([120 150 230]+128)/383;patch([0 1 1 0],[0 0 1 1],c1);patch([0 1 1 1-e 1-e 0+e],[0 0 1 1-e 0+e 0+e],c2);patch([0 0 1 1-e 0+e 0+e],[0 1 1 1-e 1-e 0+e],c3);plot([0 1 1 0 0],[0 0 1 1 0]);disp('b');
  netsum : Sum  Inputs=2  InputSameDT=on  SaturateOnIntegerOverflow=on  OutDataTypeStr=Inherit: Same as first input
      mask Display: e = 0.06;c1 = [120 150 230]/255;c2 = ([120 150 230]+0)/383;c3 = ([120 150 230]+128)/383;patch([0 1 1 0],[0 0 1 1],c1);patch([0 1 1 1-e 1-e 0+e],[0 0 1 1-e 0+e 0+e],c2);patch([0 0 1 1-e 0+e 0+e],[0 1 1 1-e 1-e 0+e],c3);plot([0 1 1 0 0],[0 0 1 1 0]);disp('+');
  purelin : neural/Transfer Functions/purelin
  "a{2}" : Outport  InitialOutput=[0;0]
      mask Display: e = 0.06;c1 = [120 230 180]/255;c2 = ([120 230 180]+0)/(256+128);c3 = ([120 230 180]+128)/(256+128);patch([0 1 1 0],[0 0 1 1],c1);patch([0 1 1 1-e 1-e 0+e],[0 0 1 1-e 0+e 0+e],c2);patch([0 0 1 1-e 0+e 0+e],[0 1 1 1-e 1-e 0+e],c3);plot([0 1 1 0 0],[0 0 1 1 0]);
  wires:
  "a{1} "/1 -> Delays 1/1("p{2}")
  Delays 1/1("pd{2,1}") -> "LW{2,1}"/1("ad{2,1}")
  "LW{2,1}"/1("lz{2,1}") -> netsum/1
  "b{2}"/1 -> netsum/2
  netsum/1 -> purelin/1
  purelin/1 -> "a{2}"/1
